simulink model "raspberrypi_ethercat_master"  (R2018b)
settings: Solver=FixedStepDiscrete  StartTime=0.0  StopTime=100  FixedStep=0.05  RelTol=1e-3  EnableMultiTasking=on
settings Model: FPTRunName=Active  ExtModeTrigDuration=2  Creator=ihout  LastModifiedBy=ihout
settings SolverCC: PositivePriorityOrder=on
settings DataIOCC: LimitDataPoints=on  MaxDataPoints=5000  SaveFormat=StructureWithTime  LoggingFileName=raspberrypi_ethercat_master.mat
settings OptimizationCC: ExpressionDepthLimit=2147483647  LifeSpan=Inf  MaxStackSize=64  SimCompilerOptimization=on
settings DebuggingCC: UnderspecifiedInitializationDetection=Classic  MergeDetectMultiDrivingBlocksExec=none  FcnCallInpInsideContextMsg=warning  AllowSymbolicDim=off  StateNameClashWarn=warning  SFUnexpectedBacktrackingDiag=warning  SFNoUnconditionalDefaultTransitionDiag=warning  SFExecutionAtInitializationDiag=none
settings HardwareCC: ProdBitPerPointer=32  ProdBitPerSizeT=32  ProdBitPerPtrDiffT=32  ProdLargestAtomicInteger=Long  ProdLargestAtomicFloat=Double  ProdWordSize=32  ProdHWDeviceType=ARM Compatible->ARM Cortex  UseEmbeddedCoderFeatures=off  UseSimulinkCoderFeatures=off
settings ModelReferenceCC: PropagateSignalLabelsOutOfModel=off
settings SFSimCC: SimUseLocalCustomCode=off
settings RTWCC: SystemTargetFile=ert.tlc  HardwareBoard=Raspberry Pi  TemplateMakefile=ert_default_tmf  GenerateReport=on  RTWVerbose=off  RTWUseLocalCustomCode=off  Toolchain=GNU GCC Raspberry Pi  BuildConfiguration=Faster Runs  LaunchReport=on
settings CodeAppCC: ForceParamTrailComments=on  OperatorAnnotations=on  StateflowObjectComments=on  MATLABSourceComments=on
settings ERTTargetCC: MultiwordLength=2048  ERTCustomFileBanners=off  SupportContinuousTime=on  SupportNonInlinedSFcns=on  RemoveResetFunc=off  SupportVariableSizeSignals=on  ModelStepFunctionPrototypeControlCompliant=off
settings ConfigComp: CovMetricSettings=dw  CovHtmlReporting=on  CovSaveCumulativeToWorkspaceVar=on  CovSaveSingleToWorkspaceVar=on  CovExternalEMLEnable=off  CovSFcnEnable=off

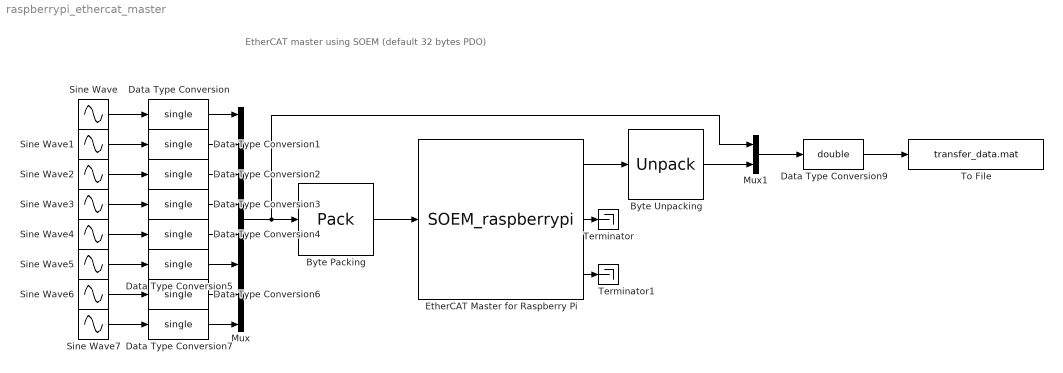
== system raspberrypi_ethercat_master ==
  note: EtherCAT master using SOEM (default 32 bytes PDO)
  Byte Packing : S-Function  InitFcn=try, set_param(gcb,'FunctionName','Pack'), end  FunctionName=Pack  SFunctionModules=Pack_wrapper  SFunctionDeploymentMode=off  EnableBusSupport=off  mask(S-Function Builder){}
      mask help: Simulink:masks:SFunctionBuilder_MD
      mask init:
      | val = [[.9  0.75 0.75 1 1 .9 .9 1]',[1 1 0.75 0.75 .9 .9 1 .9]'];try , sys = get_param(gcb,'SfunBuilderFcnName');if isempty(sys), sys = get_param(gcb,'FunctionName'); end,catch, sys = get_param(gcb,'FunctionName'); end
      settings: CopyFcn=set_param(gcbh,'LinkStatus','none')  PreSaveFcn=try, set_param(gcb,'FunctionName','Pack'), end  OpenFcn=sfunctionwizard(gcbh)
      mask Display: plot(val(:,1),val(:,2)),disp(sys), port_label('input',1,'u'), port_label('output',1,'y')
  Byte Unpacking : S-Function  InitFcn=try, set_param(gcb,'FunctionName','Unpack'), end  FunctionName=Unpack  SFunctionModules=Unpack_wrapper  SFunctionDeploymentMode=off  EnableBusSupport=off  mask(S-Function Builder){}
      mask help: Simulink:masks:SFunctionBuilder_MD
      mask init: same as raspberrypi_ethercat_master/Byte Packing
      settings: CopyFcn=set_param(gcbh,'LinkStatus','none')  PreSaveFcn=try, set_param(gcb,'FunctionName','Unpack'), end  OpenFcn=sfunctionwizard(gcbh)
      mask Display: plot(val(:,1),val(:,2)),disp(sys), port_label('input',1,'u'), port_label('output',1,'y')
  Data Type Conversion{,1..7} (8 alike) : DataTypeConversion  OutDataTypeStr=single
  Data Type Conversion9 : DataTypeConversion  OutDataTypeStr=double
  EtherCAT Master for Raspberry Pi : S-Function  InitFcn=try, set_param(gcb,'FunctionName','SOEM_raspberrypi'), end  FunctionName=SOEM_raspberrypi  Parameters=uint32(2)  SFunctionModules=SOEM_raspberrypi_wrapper  SFunctionDeploymentMode=off  EnableBusSupport=off  mask(S-Function Builder){}
      mask init: same as raspberrypi_ethercat_master/Byte Packing
      settings: CopyFcn=set_param(gcbh,'LinkStatus','none')  PreSaveFcn=try, set_param(gcb,'FunctionName','SOEM_raspberrypi'), end  OpenFcn=sfunctionwizard(gcbh)
      mask Display: plot(val(:,1),val(:,2)),disp(sys), port_label('input',1,'TxPdo'), port_label('output',1,'RxPdo'), port_label('output',2,'State'), port_label('output',3,'DCtime')
  Mux : Mux  Inputs=8
  Mux1 : Mux  Inputs=2
  Sine Wave : Sin  SineType=Sample based  Samples=20  SampleTime=0.05
  Sine Wave1 : Sin  SineType=Sample based  Bias=1  Samples=20  SampleTime=0.05
  Sine Wave2 : Sin  SineType=Sample based  Bias=2  Samples=20  SampleTime=0.05
  Sine Wave3 : Sin  SineType=Sample based  Bias=3  Samples=20  SampleTime=0.05
  Sine Wave4 : Sin  SineType=Sample based  Bias=4  Samples=20  SampleTime=0.05
  Sine Wave5 : Sin  SineType=Sample based  Bias=5  Samples=20  SampleTime=0.05
  Sine Wave6 : Sin  SineType=Sample based  Bias=6  Samples=20  SampleTime=0.05
  Sine Wave7 : Sin  SineType=Sample based  Bias=7  Samples=20  SampleTime=0.05
  Terminator : Terminator
  Terminator1 : Terminator
  To File : ToFile  Filename=transfer_data.mat  MatrixName=dataTransfer
  wires:
  Sine Wave6/1 -> Data Type Conversion6/1
  Data Type Conversion3/1 -> Mux/4
  Data Type Conversion7/1 -> Mux/8
  Data Type Conversion5/1 -> Mux/6
  Data Type Conversion1/1 -> Mux/2
  Sine Wave7/1 -> Data Type Conversion7/1
  Data Type Conversion2/1 -> Mux/3
  Sine Wave5/1 -> Data Type Conversion5/1
  Data Type Conversion6/1 -> Mux/7
  Byte Packing/1 -> EtherCAT Master for Raspberry Pi/1
  Data Type Conversion4/1 -> Mux/5
  Sine Wave1/1 -> Data Type Conversion1/1
  Mux/1 -> Mux1/1, Byte Packing/1
  Data Type Conversion/1 -> Mux/1
  Sine Wave3/1 -> Data Type Conversion3/1
  Sine Wave2/1 -> Data Type Conversion2/1
  EtherCAT Master for Raspberry Pi/1 -> Byte Unpacking/1
  Sine Wave/1 -> Data Type Conversion/1
  Sine Wave4/1 -> Data Type Conversion4/1
  Mux1/1 -> Data Type Conversion9/1
  Byte Unpacking/1 -> Mux1/2
  Data Type Conversion9/1 -> To File/1
  EtherCAT Master for Raspberry Pi/2 -> Terminator/1
  EtherCAT Master for Raspberry Pi/3 -> Terminator1/1
